simulink model "TVLQR_dist_sim"  (R2024b)
settings: Solver=FixedStepDiscrete  StartTime=0.0  StopTime=5690*100  FixedStep=1  RelTol=1e-3
values from neighbouring files (symbols this model uses):
  Ad = sys_d.A    [TVLQR2.m]    (also in TVLQR_dist.m)
  Bd = sys_d.B    [TVLQR2.m]    (also in TVLQR_dist.m)
  Cd = sys_d.C    [TVLQR2.m]    (also in TVLQR_dist.m)
  Dd = sys_d.D    [TVLQR2.m]    (also in TVLQR_dist.m)
undefined symbols (not defined in the file or in its folder): DiscIntNeverNeededParam, Pss_aug_bot, R_inv
settings Model: Creator=zalak  LastModifiedBy=zalak

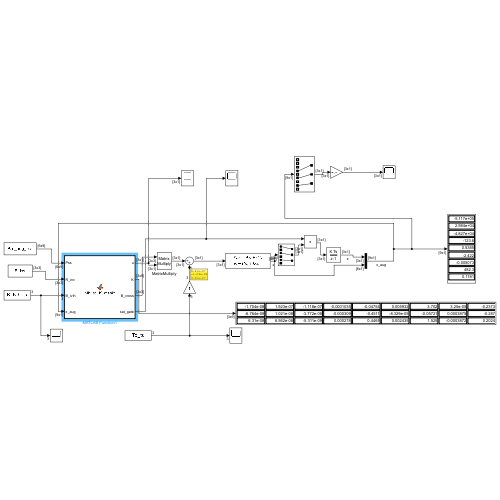
[thumbnail: Simulink's stored preview of the top-level diagram]
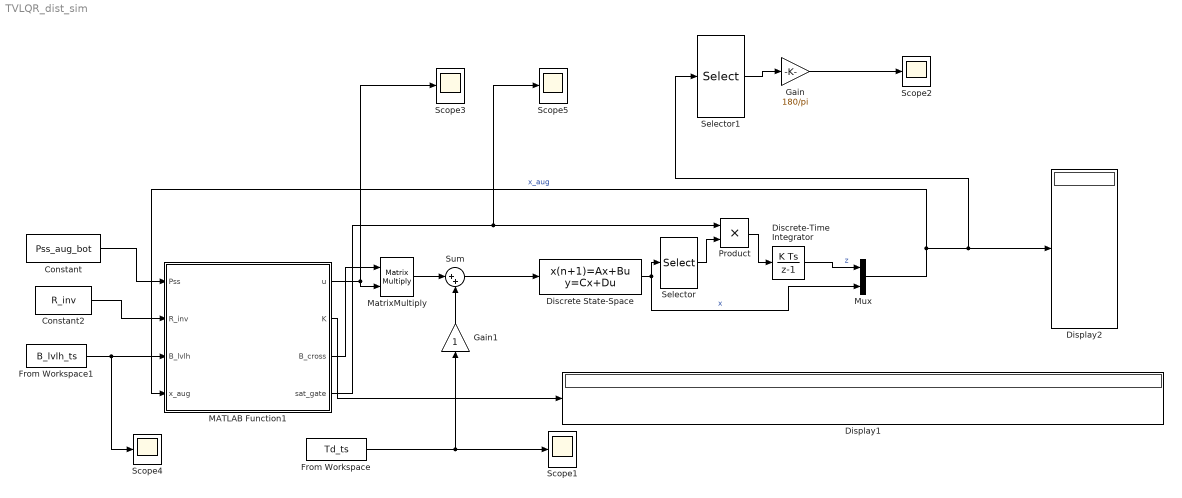
== system TVLQR_dist_sim ==
  Constant : Constant  Value=Pss_aug_bot
  Constant2 : Constant  Value=R_inv
  Discrete State-Space : DiscreteStateSpace  A=Ad  B=Bd  C=Cd  D=Dd  InitialCondition=[30*pi/180;0;30*pi/180;0;30*pi/180;0]
  Discrete-Time Integrator : DiscreteIntegrator  SampleTime=-1  ICPrevOutput=DiscIntNeverNeededParam  ICPrevScaledInput=DiscIntNeverNeededParam
  Display1 : Display
  Display2 : Display
  From Workspace : FromWorkspace  VariableName=Td_ts
  From Workspace1 : FromWorkspace  VariableName=B_lvlh_ts  SampleTime=1
  Gain : Gain  Gain=180/pi
  Gain1 : Gain
  MATLAB Function1 : MATLAB Function  TreatAsAtomicUnit=on
  MatrixMultiply : Product  Multiplication=Matrix(*)
  Mux : Mux  Inputs=2
  Product : Product
  Scope{1..5} (5 alike) : Scope
  Selector : Selector  InputPortWidth=6  IndexOptions=Index vector (dialog)  Indices=[1 3 5]  OutputSizes=1
  Selector1 : Selector  InputPortWidth=9  IndexOptions=Index vector (dialog)  Indices=[4 6 8]  OutputSizes=1
  Sum : Sum  Inputs=|++
  wires:
  Gain/1 -> Scope2/1
  From Workspace1/1 -> Scope4/1, MATLAB Function1/3(B_lvlh)
  Constant2/1 -> MATLAB Function1/2(R_inv)
  MATLAB Function1/2(K) -> Display1/1
  MATLAB Function1/1(u) -> MatrixMultiply/2, Scope3/1
  MATLAB Function1/3(B_cross) -> MatrixMultiply/1
  MatrixMultiply/1 -> Sum/1
  From Workspace/1 -> Gain1/1, Scope1/1
  Sum/1 -> Discrete State-Space/1
  Constant/1 -> MATLAB Function1/1(Pss)
  Discrete-Time Integrator/1 -> Mux/1  "z"
  Mux/1 -> MATLAB Function1/4(x_aug), Selector1/1, Display2/1  "x_aug"
  Discrete State-Space/1 -> Selector/1, Mux/2  "x"
  Gain1/1 -> Sum/2
  Selector1/1 -> Gain/1
  MATLAB Function1/4(sat_gate) -> Scope5/1, Product/1
  Selector/1 -> Product/2
  Product/1 -> Discrete-Time Integrator/1

== matlab function TVLQR_dist_sim/MATLAB Function1 ==
  data: Pss input; R_inv input; B_lvlh input; x_aug input; u output; K output; B_cross output; sat_gate output
function [u, K, B_cross, sat_gate] = lvlh_to_K_matrix(Pss, R_inv, B_lvlh, x_aug)
%   x_aug (9×1) = [z (3×1); x (6×1)]
%   Pss is Pss_aug_bot (6×9, constant pass-through)
mass = 2.0;  Lx = 0.226;  Ly = 0.100;  Lz = 0.100;
Ix = (1/12)*mass*(Ly^2+Lz^2);
Iy = (1/12)*mass*(Lx^2+Lz^2);
Iz = (1/12)*mass*(Lx^2+Ly^2);

alpha0   = 7.9991;       % alpha_opt_aug from Floquet sweep
m_max_hw = 0.2;             % hardware dipole limit [A·m^2]

% Extract attitude from augmented state
x   = x_aug(4:9);
phi = x(1); theta = x(3); psi = x(5);

Rx = [1,0,0; 0,cos(phi),sin(phi); 0,-sin(phi),cos(phi)];
Ry = [cos(theta),0,-sin(theta); 0,1,0; sin(theta),0,cos(theta)];
Rz = [cos(psi),sin(psi),0; -sin(psi),cos(psi),0; 0,0,1];

B_body = Rz*Ry*Rx * B_lvlh(:);
bx = B_body(1); by = B_body(2); bz = B_body(3);

B_cross = [0,bz,-by; -bz,0,bx; by,-bx,0];

B_tv = zeros(6,3);
B_tv(2,:) = B_cross(1,:)/Ix;
B_tv(4,:) = B_cross(2,:)/Iy;
B_tv(6,:) = B_cross(3,:)/Iz;

% Compute nominal control (Psiaki eq. 22a)
K     = alpha0 * R_inv * (B_tv' * Pss);     % 3×9 gain
u_nom = -K * x_aug;                          % 3×1 nominal dipole command

beta = max(abs(u_nom) / m_max_hw);
if beta > 1
    u = u_nom / beta;
    sat_gate = 0;        % freeze integrator
else
    u = u_nom;
    sat_gate = 1;        % allow integration
end

end
